simulink model "FuzzyPID_Quadrotor"  (R2025a)
settings: Solver=ode8  StartTime=0.0  StopTime=40  FixedStep=0.002  RelTol=1e-3
undefined symbols (not defined in the file): b, d, g, Ir, Ixx, Iyy, Izz, k_phi, Ki, Kp, kx, l, m
libraries: fuzblock x6, slpidlib x6, simulink x2
(part 2 of 2)

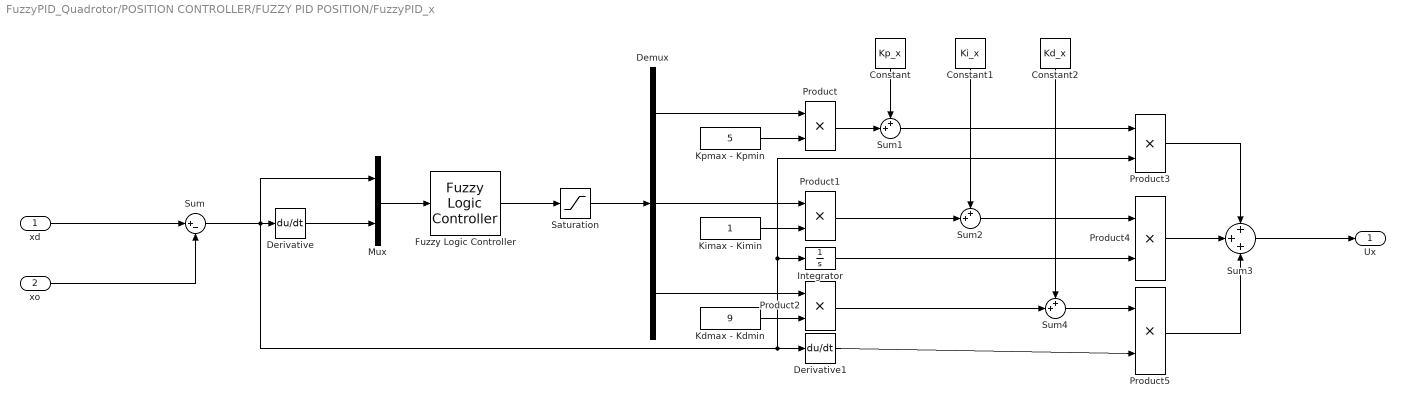
== system FuzzyPID_Quadrotor/POSITION CONTROLLER/FUZZY PID POSITION/FuzzyPID_x ==
  xd : Inport
  xo : Inport  Port=2
  Constant : Constant  Value=Kp_x
  Constant1 : Constant  Value=Ki_x
  Constant2 : Constant  Value=Kd_x
  Demux : Demux  Outputs=3
  Derivative : Derivative
  Derivative1 : Derivative
  Fuzzy Logic Controller : fuzblock/Fuzzy Logic  Controller  FIS='FuzzyPID_Controller.fis'  OutputSampleNumber=101  DataType=double  UseLookupTable=off  NumBreakpoints=10  FuzzifiedInputs=off  RuleFiringStrengths=off  RuleOutputs=off  AggregatedOutputs=off  SimulateUsing=Interpreted execution  OutOfRangeInputValueMessage=warning  NoRuleFiredMessage=warning  EmptyOutputFuzzySetMessage=warning
  Integrator : Integrator
  Kdmax - Kdmin : Constant  Value=9
  Kimax - Kimin : Constant
  Kpmax - Kpmin : Constant  Value=5
  Mux : Mux  Inputs=2
  Product{,1..5} (6 alike) : Product
  Saturation : Saturate
  Sum : Sum  Inputs=|+-
  Sum1 : Sum  Inputs=++|
  Sum2 : Sum  Inputs=++|
  Sum3 : Sum  Inputs=+++
  Sum4 : Sum  Inputs=++|
  Ux : Outport
  wires:
  Product1/1 -> Sum2/2
  Demux/1 -> Product/1
  Kpmax - Kpmin/1 -> Product/2
  Fuzzy Logic Controller/1 -> Saturation/1
  Kimax - Kimin/1 -> Product1/2
  Constant/1 -> Sum1/1
  Product/1 -> Sum1/2
  Derivative1/1 -> Product5/2
  Integrator/1 -> Product4/2
  Sum/1 -> Mux/1, Product3/2, Integrator/1, Derivative1/1, Derivative/1
  Product4/1 -> Sum3/2
  Sum4/1 -> Product5/1
  Kdmax - Kdmin/1 -> Product2/2
  Sum2/1 -> Product4/1
  Demux/3 -> Product2/1
  Sum3/1 -> Ux/1
  Derivative/1 -> Mux/2
  Constant2/1 -> Sum4/1
  Constant1/1 -> Sum2/1
  Product3/1 -> Sum3/1
  Product5/1 -> Sum3/3
  Mux/1 -> Fuzzy Logic Controller/1
  Product2/1 -> Sum4/2
  Sum1/1 -> Product3/1
  Demux/2 -> Product1/1
  Saturation/1 -> Demux/1
  xo/1 -> Sum/2
  xd/1 -> Sum/1

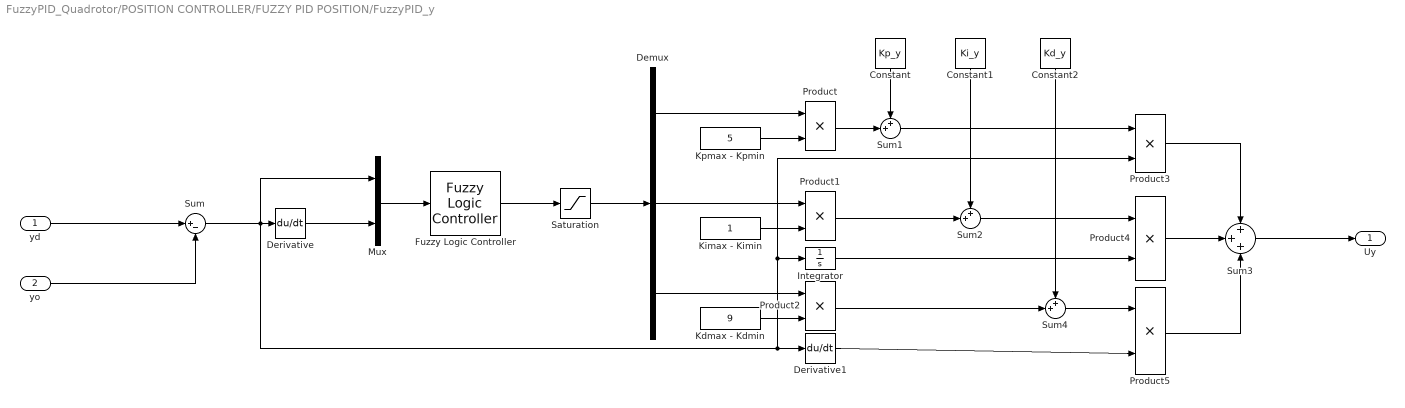
== system FuzzyPID_Quadrotor/POSITION CONTROLLER/FUZZY PID POSITION/FuzzyPID_y ==
  yd : Inport
  yo : Inport  Port=2
  Constant : Constant  Value=Kp_y
  Constant1 : Constant  Value=Ki_y
  Constant2 : Constant  Value=Kd_y
  Demux : Demux  Outputs=3
  Derivative : Derivative
  Derivative1 : Derivative
  Fuzzy Logic Controller : fuzblock/Fuzzy Logic  Controller  FIS='FuzzyPID_Controller.fis'  OutputSampleNumber=101  DataType=double  UseLookupTable=off  NumBreakpoints=10  FuzzifiedInputs=off  RuleFiringStrengths=off  RuleOutputs=off  AggregatedOutputs=off  SimulateUsing=Interpreted execution  OutOfRangeInputValueMessage=warning  NoRuleFiredMessage=warning  EmptyOutputFuzzySetMessage=warning
  Integrator : Integrator
  Kdmax - Kdmin : Constant  Value=9
  Kimax - Kimin : Constant
  Kpmax - Kpmin : Constant  Value=5
  Mux : Mux  Inputs=2
  Product{,1..5} (6 alike) : Product
  Saturation : Saturate
  Sum : Sum  Inputs=|+-
  Sum1 : Sum  Inputs=++|
  Sum2 : Sum  Inputs=++|
  Sum3 : Sum  Inputs=+++
  Sum4 : Sum  Inputs=++|
  Uy : Outport
  wires:
  yd/1 -> Sum/1
  yo/1 -> Sum/2
  Saturation/1 -> Demux/1
  Demux/2 -> Product1/1
  Sum1/1 -> Product3/1
  Product2/1 -> Sum4/2
  Mux/1 -> Fuzzy Logic Controller/1
  Product5/1 -> Sum3/3
  Product3/1 -> Sum3/1
  Constant1/1 -> Sum2/1
  Constant2/1 -> Sum4/1
  Derivative/1 -> Mux/2
  Sum3/1 -> Uy/1
  Demux/3 -> Product2/1
  Sum2/1 -> Product4/1
  Kdmax - Kdmin/1 -> Product2/2
  Sum4/1 -> Product5/1
  Product4/1 -> Sum3/2
  Sum/1 -> Derivative/1, Derivative1/1, Integrator/1, Product3/2, Mux/1
  Integrator/1 -> Product4/2
  Derivative1/1 -> Product5/2
  Product/1 -> Sum1/2
  Constant/1 -> Sum1/1
  Kimax - Kimin/1 -> Product1/2
  Fuzzy Logic Controller/1 -> Saturation/1
  Kpmax - Kpmin/1 -> Product/2
  Demux/1 -> Product/1
  Product1/1 -> Sum2/2

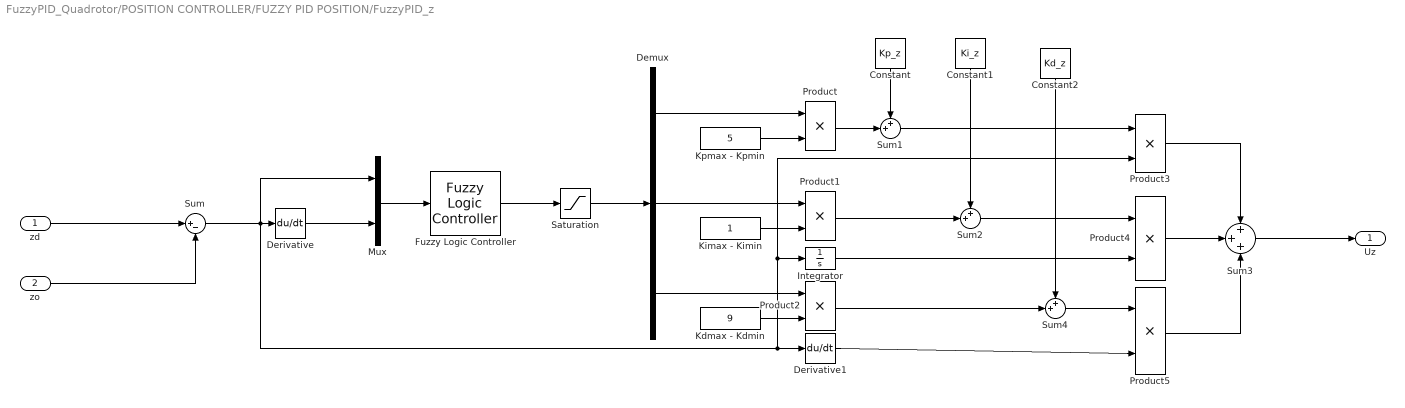
== system FuzzyPID_Quadrotor/POSITION CONTROLLER/FUZZY PID POSITION/FuzzyPID_z ==
  zd : Inport
  zo : Inport  Port=2
  Constant : Constant  Value=Kp_z
  Constant1 : Constant  Value=Ki_z
  Constant2 : Constant  Value=Kd_z
  Demux : Demux  Outputs=3
  Derivative : Derivative
  Derivative1 : Derivative
  Fuzzy Logic Controller : fuzblock/Fuzzy Logic  Controller  FIS='FuzzyPID_Controller.fis'  OutputSampleNumber=101  DataType=double  UseLookupTable=off  NumBreakpoints=10  FuzzifiedInputs=off  RuleFiringStrengths=off  RuleOutputs=off  AggregatedOutputs=off  SimulateUsing=Interpreted execution  OutOfRangeInputValueMessage=warning  NoRuleFiredMessage=warning  EmptyOutputFuzzySetMessage=warning
  Integrator : Integrator
  Kdmax - Kdmin : Constant  Value=9
  Kimax - Kimin : Constant
  Kpmax - Kpmin : Constant  Value=5
  Mux : Mux  Inputs=2
  Product{,1..5} (6 alike) : Product
  Saturation : Saturate
  Sum : Sum  Inputs=|+-
  Sum1 : Sum  Inputs=++|
  Sum2 : Sum  Inputs=++|
  Sum3 : Sum  Inputs=+++
  Sum4 : Sum  Inputs=++|
  Uz : Outport
  wires:
  Product1/1 -> Sum2/2
  Demux/1 -> Product/1
  Kpmax - Kpmin/1 -> Product/2
  Fuzzy Logic Controller/1 -> Saturation/1
  Kimax - Kimin/1 -> Product1/2
  Constant/1 -> Sum1/1
  Product/1 -> Sum1/2
  Derivative1/1 -> Product5/2
  Integrator/1 -> Product4/2
  Sum/1 -> Mux/1, Product3/2, Integrator/1, Derivative1/1, Derivative/1
  Product4/1 -> Sum3/2
  Sum4/1 -> Product5/1
  Kdmax - Kdmin/1 -> Product2/2
  Sum2/1 -> Product4/1
  Demux/3 -> Product2/1
  Sum3/1 -> Uz/1
  Derivative/1 -> Mux/2
  Constant2/1 -> Sum4/1
  Constant1/1 -> Sum2/1
  Product3/1 -> Sum3/1
  Product5/1 -> Sum3/3
  Mux/1 -> Fuzzy Logic Controller/1
  Product2/1 -> Sum4/2
  Sum1/1 -> Product3/1
  Demux/2 -> Product1/1
  Saturation/1 -> Demux/1
  zo/1 -> Sum/2
  zd/1 -> Sum/1

== system FuzzyPID_Quadrotor/POSITION CONTROLLER/Subsystem/Roll  ==
  Ux : Inport
  Uy : Inport  Port=2
  Uz : Inport  Port=3
  ψd : Inport  Port=4
  Add : Sum
  Asin : Trigonometry  Operator=asin
  Constant : Constant  Value=m*g
  Cos : Trigonometry  Operator=cos
  Fcn : Fcn  Expr=u^2
  Fcn1 : Fcn  Expr=u^2
  Fcn2 : Fcn  Expr=u^2
  Product : Product
  Product1 : Product
  Product2 : Product  Inputs=*/
  Sin : Trigonometry
  Sqrt : Sqrt
  Sum : Sum  Inputs=+++
  Sum1 : Sum  Inputs=+-
  ϕd : Outport
  wires:
  Ux/1 -> Product/2, Fcn/1
  Fcn1/1 -> Sum/2
  Uy/1 -> Product1/2, Fcn1/1
  Sqrt/1 -> Product2/2
  Add/1 -> Fcn2/1
  Fcn2/1 -> Sum/3
  Uz/1 -> Add/1
  Fcn/1 -> Sum/1
  Sum/1 -> Sqrt/1
  Constant/1 -> Add/2
  ψd/1 -> Sin/1, Cos/1
  Sin/1 -> Product/1
  Cos/1 -> Product1/1
  Product/1 -> Sum1/1
  Product1/1 -> Sum1/2
  Sum1/1 -> Product2/1
  Product2/1 -> Asin/1
  Asin/1 -> ϕd/1

== system FuzzyPID_Quadrotor/POSITION CONTROLLER/Subsystem/Theta ==
  Ux : Inport
  Uy : Inport  Port=2
  Uz : Inport  Port=3
  ψd : Inport  Port=4
  Add : Sum
  Atan : Trigonometry  Operator=atan
  Constant : Constant  Value=m*g
  Cos : Trigonometry  Operator=cos
  Product : Product
  Product1 : Product
  Product2 : Product  Inputs=*/
  Sin : Trigonometry
  Sum : Sum
  θd : Outport
  wires:
  ψd/1 -> Cos/1, Sin/1
  Cos/1 -> Product/1
  Ux/1 -> Product/2
  Uy/1 -> Product1/2
  Sin/1 -> Product1/1
  Product/1 -> Sum/1
  Product1/1 -> Sum/2
  Uz/1 -> Add/1
  Constant/1 -> Add/2
  Sum/1 -> Product2/1
  Add/1 -> Product2/2
  Product2/1 -> Atan/1
  Atan/1 -> θd/1

== system FuzzyPID_Quadrotor/POSITION CONTROLLER/Subsystem/Thrust ==
  Ux : Inport
  Uy : Inport  Port=2
  Uz : Inport  Port=3
  Add : Sum
  Constant : Constant  Value=m*g
  Fcn : Fcn  Expr=u^2
  Fcn1 : Fcn  Expr=u^2
  Fcn2 : Fcn  Expr=u^2
  Sqrt : Sqrt
  Sum : Sum  Inputs=+++
  U1 : Outport
  wires:
  Constant/1 -> Add/2
  Sum/1 -> Sqrt/1
  Fcn/1 -> Sum/1
  Uz/1 -> Add/1
  Fcn2/1 -> Sum/3
  Add/1 -> Fcn2/1
  Uy/1 -> Fcn1/1
  Fcn1/1 -> Sum/2
  Ux/1 -> Fcn/1
  Sqrt/1 -> U1/1

== matlab function FuzzyPID_Quadrotor/SquareTrajectory/MATLAB Function ==
  data: u input; yd output
function yd = fcn(u)
%#codegen
yd = 0;
if u < 10
    yd = u;
end
if u>=10 && u<20
    yd = 10;
end
if u>=20 && u<30
    yd = 30 - u;
end
if u>=30 && u<40
    yd = 0;
end

== matlab function FuzzyPID_Quadrotor/SquareTrajectory/MATLAB Function1 ==
  data: u input; xd output
function xd = fcn(u)
%#codegen
xd = 0;
if u < 10
    xd = 0;
end
if u>=10 && u<20
    xd = -10 + u;
end
if u>=20 && u<30
    xd = 10;
end
if u>=30 && u<40
    xd = 40 - u;
end

== matlab function FuzzyPID_Quadrotor/MATLAB Function1 ==
  data: u input; zd output
function zd = fcn(u)
%#codegen
zd=6;
